simulink model "GalvoModel_v31_19082014"  (R2013a)
settings: Solver=ode45  StartTime=0.0  StopTime=30e-3  RelTol=1e-3
model workspace (MAT data in the model file):
  Var = 0
libraries: simulink x1
settings Model: BufferReuse=off  Creator=mainster  LastModifiedBy=mainster
settings OptimizationCC: InlineParams=on  BufferReuse=off
settings DebuggingCC: SolverPrmCheckMsg=none  InitInArrayFormatMsg=none
settings ModelReferenceCC: ModelReferenceNumInstancesAllowed=Single  ModelReferenceMinAlgLoopOccurrences=on

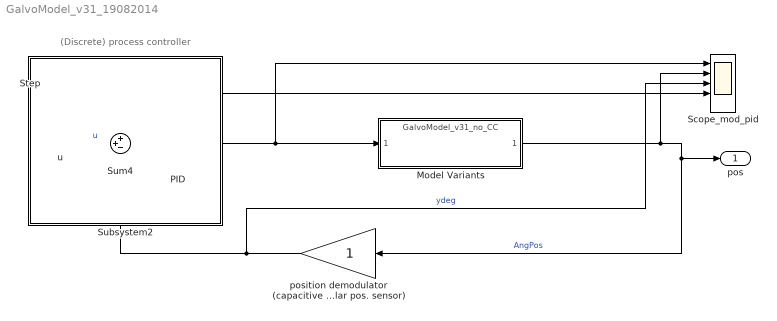
== system GalvoModel_v31_19082014 ==
  note: (Discrete) process controller
  u : Inport
  Model Variants : ModelReference  ModelNameDialog=GalvoModel_v31_no_CC.slx  SimulationMode=Normal  Variant=on  ModelReferenceVersion=1.35  CopyOfModelName=GalvoModel_v31_no_CC.slx  DefaultDataLogging=on
      settings: AttributesFormatString=%<ActiveVariant>
  PID : simulink/Continuous/PID Controller  Controller=PID  TimeDomain=Continuous-time  SampleTime=1  IntegratorMethod=Forward Euler  FilterMethod=Forward Euler  Form=Parallel  P=7.56667246001753  I=220.767682586481  D=0.0576229306626934  N=571544.823549136  InitialConditionSource=internal  InitialConditionForIntegrator=0  InitialConditionForFilter=0  ExternalReset=none  LimitOutput=on  UpperSaturationLimit=25  LowerSaturationLimit=-25  LinearizeAsGain=off  AntiWindupMode=back-calculation  Kb=1  TrackingMode=off  Kt=0  PParamMin=[]  PParamMax=[]  IParamMin=[]  IParamMax=[]  DParamMin=[]  DParamMax=[]  NParamMin=[]  NParamMax=[]  KbParamMin=[]  KbParamMax=[]  KtParamMin=[]  KtParamMax=[]  POutMin=[]  POutMax=[]  IOutMin=[]  IOutMax=[]  DOutMin=[]  DOutMax=[]  NOutMin=[]  NOutMax=[]  KbOutMin=[]  KbOutMax=[]  KtOutMin=[]  KtOutMax=[]  IntegratorOutMin=[]  IntegratorOutMax=[]  FilterOutMin=[]  FilterOutMax=[]  SumOutMin=[]  SumOutMax=[]  SumI1OutMin=[]  SumI1OutMax=[]  SumI2OutMin=[]  SumI2OutMax=[]  SumI3OutMin=[]  SumI3OutMax=[]  SumDOutMin=[]  SumDOutMax=[]  SaturationOutMin=[]  SaturationOutMax=[]  IntegratorContinuousStateAttributes=''  IntegratorStateMustResolveToSignalObject=off  IntegratorRTWStateStorageClass=Auto  FilterContinuousStateAttributes=''  FilterStateMustResolveToSignalObject=off  FilterRTWStateStorageClass=Auto
  Scope_mod_pid : Scope  NumInputPorts=5
      settings: ShowLegends=on  TimeRange=0.03  YMin=-10~0~0~-0.5~-1  YMax=30~1.5~1.5~1~1  MaxDataPoints=500000
  Step : Step  Time=1e-3  SampleTime=0
      settings: AttributesFormatString=Ampl.: %<After>
  Subsystem2 : Subsystem  mask{d=0}
      mask Display: disp('')
  Sum4 : Sum  Inputs=++-
  position demodulator (capacitive angular pos. sensor) : Gain
  pos : Outport
  wires:
  Sum4/1 -> Scope_mod_pid/4, PID/1
  Step/1 -> Sum4/1
  u/1 -> Sum4/2  "u"
  position demodulator (capacitive angular pos. sensor)/1 -> Scope_mod_pid/3, Sum4/3  "ydeg"
  Model Variants/1 -> Scope_mod_pid/2, position demodulator (capacitive angular pos. sensor)/1, pos/1  "AngPos"
  PID/1 -> Model Variants/1, Scope_mod_pid/1

== system GalvoModel_v31_19082014/Subsystem2 ==
